simulink model "Sequence_Manager"  (R2024a)
settings: Solver=ode1  StartTime=0.0  StopTime=inf  FixedStep=0.1  RelTol=1e-3
undefined symbols (not defined in the file): Angle, Axis, Battery, s
libraries: robotcorelib x6, eeGeneralControl x6, slpidlib x4
settings Model: Creator=Sasha  LastModifiedBy=Sasha

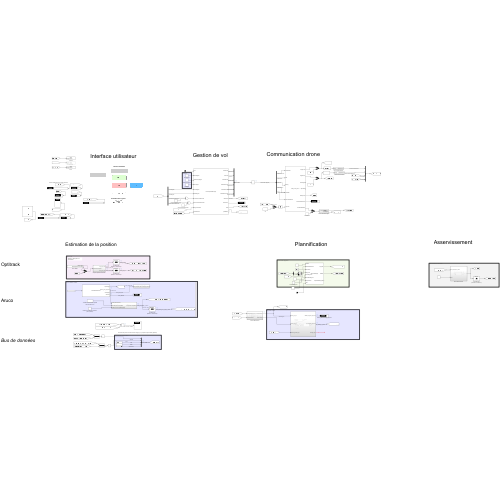
[thumbnail: Simulink's stored preview of the top-level diagram]
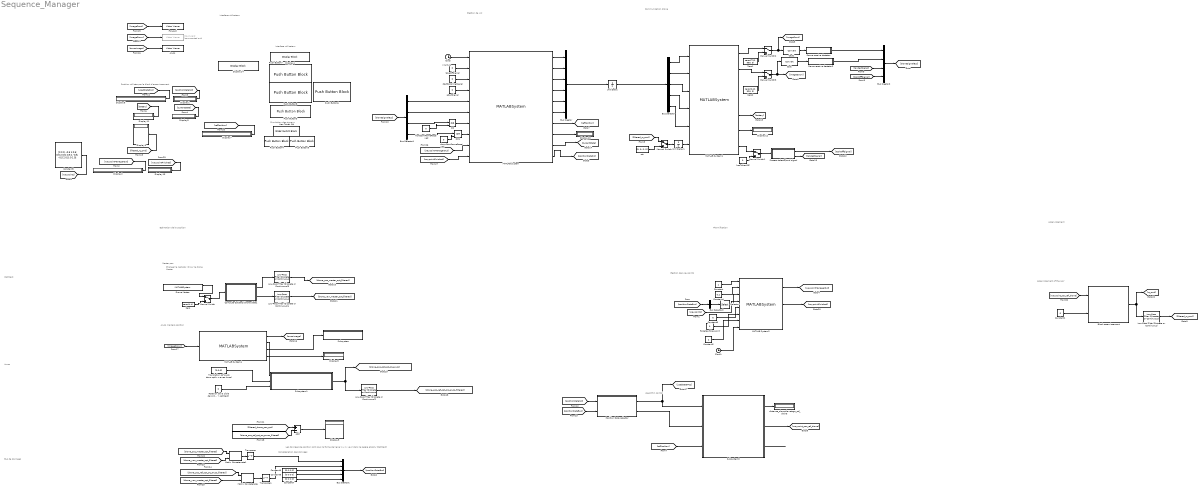
== system Sequence_Manager ==
  note: Plannification
  note: Estimation de la position
  note: Position utilisée par le block d'asservissement
  note: Gestion des waypoints
  note: Interface
  note: Concaténation des données
  note: Les données de position sont sous la forme de ligne (x,y,z, yaw) dans le repère absolu (Optitrack)
  note: Simulation des signaux
  note: Master pos
  note: Changer le rigibody ID sur le drone Master
  note: Algorithm control
  note: Interface utilisateur
  note: Aruco markers position
  note: Optitrack
  note: Aruco
  note: Bus de données
  note: Asservissement
  note: Gestion de vol
  note: Communication drone
  note: Interface utilisateur
  note: Asservissement of the UAV
  Add : Sum  Inputs=+-
  Aruco : VideoViewer  FigPos=[1259 530 247.333333333333 297.333333333333]
  "Block asservissement " : Subsystem
  Bus Creator : BusCreator  Inputs=6
  Bus Creator1 : BusCreator  Inputs=5
  Bus Creator2 : BusCreator  Inputs=4
  Bus Selector : BusSelector  OutputSignals=enableVideoCmd,takeOffCmd,landCmd,enableRcCmd,videoDirectionCmd
  Bus Selector1 : BusSelector  OutputSignals=tookOffSignal,landedSignal,frontCamFrameReceived,downCamFrameReceived
  Bus Selector2 : BusSelector  OutputSignals=Optitrack
  Cast : DataTypeConversion  SaturateOnIntegerOverflow=off  RndMeth=Floor
  Cast1 : DataTypeConversion  SaturateOnIntegerOverflow=off  RndMeth=Floor
  Clock : Clock
  Clock1 : Clock
  Compute Optitrack Drone data1 : Subsystem
  Constant : Constant
  Constant1 : Constant  Value=0
  Constant2 : Constant  Value=2
  Constant4 : Constant  Value=0.2
  Constant5 : Constant  Value="[0 0 0; -0.5 1 0.5;  0.5 2 0.5; 0.5 1 -0.5; -0.5 2 0.5; 0 1 0]"
  Constant6 : Constant  Value=6
  Constant7 : Constant  Value=[0 0 0 0]
  Constant8 : Constant  Value=[0 0 0 0]
  Constant9 : Constant  Value=[0 0 0 0]
  Display{1..3,5..13} (12 alike) : Display
  Display14 : DisplayBlock  LabelPosition=Hide  Format=Custom  Transparency=1  FormatString=Battery : %s/100
  Display4 : DisplayBlock  LabelPosition=Hide  Format=Integer  Transparency=1  FormatString=%s
  Downward : VideoViewer  Commented=on  FigPos=[1261.66666666667 919.333333333333 248 307.333333333333]
  Drone Master : MATLABSystem  System=OptilinkSystem  HostIP=10.147.125.15  ClientIP=10.147.125.17  RigidbodyID=1  SimulateUsing=Interpreted execution
      mask Type: OptilinkSystem
      mask Display:
      | disp('OptilinkSystem');
      | port_label('output',1,'Drones data');
      | port_label('output',2,'Connected');
  Forward : VideoViewer  FigPos=[616.333333333333 756 875.333333333333 522.666666666667]
  Frame receive dectetor : Subsystem
  Frame receive dectetor2 : Subsystem
  Has Taken Off : SliderSwitchBlock
      settings: Values={{'Off', 'On'}, [0 1]}
  Low-Pass Filter (Discrete or Continuous) : eeGeneralControl/Low-Pass Filter (Discrete or Continuous)  K=1  T=1  B=inf  A=-inf  init_option=Inherited from block input  x0=0  Ts=-1
  Low-Pass Filter (Discrete or Continuous)2 : eeGeneralControl/Low-Pass Filter (Discrete or Continuous)  K=1  T=1.5  B=inf  A=-inf  init_option=Inherited from block input  x0=0  Ts=-1
  Low-Pass Filter (Discrete or Continuous)4 : eeGeneralControl/Low-Pass Filter (Discrete or Continuous)  K=1  T=1.5  B=inf  A=-inf  init_option=Inherited from block input  x0=0  Ts=-1
  Low-Pass Filter (Discrete or Continuous)5 : eeGeneralControl/Low-Pass Filter (Discrete or Continuous)  K=1  T=1.5  B=inf  A=-inf  init_option=Inherited from block input  x0=0  Ts=-1
  MATLAB System : MATLABSystem  System=DroneSequenceManager  HomePosition=[ 0, 1.5, 0 ]  SimulateUsing=Code generation
      mask Type: DroneSequenceManager
      mask Display:
      | disp('DroneSequenceManager');
      | port_label('input',1,'time');
      | port_label('input',2,'takeOffSignal');
      | port_label('input',3,'startPatrolingSignal');
      | port_label('input',4,'abortSignal');
      | port_label('input',5,'tookOffSignal');
      | port_label('input',6,'landedSignal');
      | port_label('input',7,'frontCamFrameReceived');
      | port_label('input',8,'downCamFrameReceived');
      | port_label('input',9,'waypointToFollow');
      | port_label('input',10,'finishedFollow');
      | port_label('output',1,'takeoffCmd');
      | port_label('output',2,'landCmd');
      | port_label('output',3,'enableRcCmd');
      | port_label('output',4,'enableVideoCmd');
      | port_label('output',5,'enableSlamCmd');
      | port_label('output',6,'videoDirectionCmd');
      | port_label('output',7,'refPosition');
      | port_label('output',8,'timeCounter');
      | port_label('output',9,'state');
      | port_label('output',10,'posDataSrc');
  MATLAB System1 : MATLABSystem  System=Tello_drone_control  droneIP=127.0.0.1  SimulateUsing=Interpreted execution
      mask Type: Tello_drone_control
      mask Display:
      | disp('Tello_drone_control');
      | port_label('input',1,'enableVideo');
      | port_label('input',2,'tkoff');
      | port_label('input',3,'landing');
      | port_label('input',4,'enableRC');
      | port_label('input',5,'cmdVideoDirection');
      | port_label('input',6,'rcspeeds');
      | port_label('output',1,'imageFront');
      | port_label('output',2,'imageDown');
      | port_label('output',3,'Eulerangles');
      | port_label('output',4,'speedXYZ');
      | port_label('output',5,'batteryLevel');
      | port_label('output',6,'currentVideoDirection');
      | port_label('output',7,'hasTakenOffStatus');
  MATLAB System2 : MATLABSystem  System=WaypointManager  SimulateUsing=Code generation
      mask Type: WaypointManager
      mask Display:
      | disp('WaypointManager');
      | port_label('input',1,'enable');
      | port_label('input',2,'lookaheadDistance');
      | port_label('input',3,'currentPos');
      | port_label('input',4,'waypoints');
      | port_label('input',5,'numWaypoints');
      | port_label('input',6,'forceNextWaypoint');
      | port_label('input',7,'requiredTime');
      | port_label('input',8,'time');
      | port_label('output',1,'waypoint');
      | port_label('output',2,'finished');
      | port_label('output',3,'elapsedTimeWaypoint');
  MATLAB System4 : MATLABSystem  System=ArucoMarkerDetection  markerSizeInMM=150  markerFamily=DICT_4X4_250  maxMarkers=1  focalLength=[222.5, 224]  principalPoint=[156 ,116]  imageSize=[240,320]  SimulateUsing=Interpreted execution
      mask Type: ArucoMarkerDetection
      mask Display:
      | disp('ArucoMarkerDetection');
      | port_label('input',1,'I');
      | port_label('output',1,'outputImage');
      | port_label('output',2,'camera_pos_ref_aruco');
      | port_label('output',3,'eulerAngles');
      | port_label('output',4,'detection');
  Manual Switch{,1..4} (5 alike) : ManualSwitch
  Matrix Concatenate : Concatenate  ConcatenateDimension=2
  Matrix Concatenate1 : Concatenate  ConcatenateDimension=2
  OR : Logic  Operator=OR  IconShape=distinctive  AllPortsSameDT=off  OutDataTypeStr=boolean
  OR1 : Logic  Operator=OR  IconShape=distinctive  AllPortsSameDT=off  OutDataTypeStr=boolean
  Position Data selector : Subsystem
  Process takeoff/land signal : Subsystem
  Push Button3 : PushButtonBlock  ButtonText=Force next waypoint  OffValue=0.000000
  Push Button4 : PushButtonBlock  ButtonText=Front cam received  OffValue=0.000000
  Push Button5 : PushButtonBlock  ButtonText=Down cam received  OffValue=0.000000
  Push Button6 : PushButtonBlock  ButtonText=Start patrol  Opacity=0.8  OffValue=0.000000
  Push Button7 : PushButtonBlock  ButtonText=Décoler  OffValue=0.000000
  Push Button8 : PushButtonBlock  ButtonText=Atterir  OffValue=0.000000
  Rotation de la cible dans Optitrack (Axe Y optitrack) : Constant  Value=0
  Selector : Selector  InputPortWidth=4  IndexOptions=Index vector (dialog)  Indices=[1 2 3]  OutputSizes=1
  Subsystem : Subsystem
  Subsystem1 : Subsystem
  Subsystem3 : Subsystem
  "Translation ref Aruco dans optitrack (dans les axes Aruco) " : Constant  Value=[0;0;0]
  Transpose : Math  Operator=transpose
  Transpose1 : Math  Operator=transpose
  Unit Delay : UnitDelay  SampleTime=-1  HasFrameUpgradeWarning=on
  Unit Delay1 : UnitDelay  InitialCondition=[0,0,0,0]  SampleTime=-1  HasFrameUpgradeWarning=on
  Zero : Constant  Value=zeros(4,4)  OutDataTypeStr=Inherit: Inherit via back propagation
  Zero1 : Constant  Value=zeros(720, 960, 3)  OutDataTypeStr=Inherit: Inherit via back propagation
  Zero2 : Constant  Value=zeros(240, 320, 3)  OutDataTypeStr=Inherit: Inherit via back propagation
  abortSignal : Constant  Value=0
  cst : Constant  Value=[0; 0; 0; 0]
  distance_slave/slavetogo_ref_drone : Display
  downCamFrameReceived : Constant  Value=0
  forceNextWaypoint : Constant  Value=0
  frontCamFrameReceived : Constant  Value=0
  hasTakenOff : Constant  Value=0
  startPatrolingSignal : Constant  Value=0
  takeOffSignal : Constant  Value=0
  wires:
  Clock/1 -> MATLAB System/1
  takeOffSignal/1 -> MATLAB System/2
  MATLAB System/6 -> Bus Creator/6  "videoDirectionCmd"
  Zero2/1 -> Manual Switch3/2
  Frame receive dectetor2/1(frameReceived) -> Bus Creator2/2  "downCamFrameReceived"
  abortSignal/1 -> MATLAB System/4
  Bus Selector1/1 -> MATLAB System/5  "<tookOffSignal>"
  Bus Selector1/2 -> MATLAB System/6  "<landedSignal>"
  MATLAB System/8 -> Display10/1
  Frame receive dectetor/1(frameReceived) -> Bus Creator2/1  "frontCamFrameReceived"
  OR/1 -> MATLAB System/7
  Bus Selector1/3 -> OR/1  "<frontCamFrameReceived>"
  frontCamFrameReceived/1 -> OR/2
  OR1/1 -> MATLAB System/8
  Bus Selector1/4 -> OR1/1  "<downCamFrameReceived>"
  downCamFrameReceived/1 -> OR1/2
  MATLAB System/1 -> Bus Creator/1  "takeOffCmd"
  MATLAB System/2 -> Bus Creator/2  "landCmd"
  MATLAB System/3 -> Bus Creator/3  "enableRcCmd"
  MATLAB System/4 -> Bus Creator/4  "enableVideoCmd"
  MATLAB System/5 -> Bus Creator/5  "enableSlamCmd"
  MATLAB System/9 -> [currentState]
  startPatrolingSignal/1 -> MATLAB System/3
  Constant9/1 -> Bus Creator1/3  "IMU"
  MATLAB System/10 -> [positionDataSrc]
  Constant4/1 -> MATLAB System2/2
  Bus Selector2/1 -> Selector/1  "<Optitrack>"
  [waypoints] -> MATLAB System2/4
  Constant6/1 -> MATLAB System2/5
  MATLAB System2/1 -> [waypointManagerOut]
  Drone Master/1 -> Manual Switch/1
  Compute Optitrack Drone data1/1(drone_pos_opt) -> Low-Pass Filter (Discrete or Continuous)5/1  "drone_pos_ref_opt"
  Low-Pass Filter (Discrete or Continuous)4/1 -> [drone_yaw_master_opt_filtered]  "drone_yaw_opt"
  Compute Optitrack Drone data1/2(drone_yaw_opt) -> Low-Pass Filter (Discrete or Continuous)4/1  "drone_yaw_ref_opt"
  Low-Pass Filter (Discrete or Continuous)5/1 -> [drone_pos_master_opt_filtered]  "drone_pos_opt"
  MATLAB System1/5 -> [battery]
  MATLAB System1/6 -> Display12/1
  Subsystem3/3(Consigne_yaw) -> ?
  Subsystem3/2(pos_waypoint_ref_drone) -> [waypoint_pos_ref_drone]  "pos_slavetogo_ref_drone"
  Position Data selector/2(Drone Yaw Opt) -> Subsystem3/2(drone_yaw_opt)
  Subsystem3/1(distance_waypoint_ref_drone) -> distance_slave/slavetogo_ref_drone/1
  [refPosition] -> Subsystem3/3(reference_position_opt)
  [filtered_rc_cmd] -> Manual Switch4/1  "filtered_rc_cmd"
  Manual Switch/1 -> Compute Optitrack Drone data1/1(Optitrack Drone TForm)
  Zero/1 -> Manual Switch/2
  Bus Creator/1 -> Unit Delay/1  "droneCmdBus"
  Bus Selector/2 -> MATLAB System1/2  "<takeOffCmd>"
  Bus Selector/3 -> MATLAB System1/3  "<landCmd>"
  Bus Selector/1 -> MATLAB System1/1  "<enableVideoCmd>"
  Bus Selector/4 -> MATLAB System1/4  "<enableRcCmd>"
  Bus Creator1/1 -> [positionDataBus]  "positionDataBus"
  Bus Selector/5 -> MATLAB System1/5  "<videoDirectionCmd>"
  Constant7/1 -> Bus Creator1/5  "SensorFusion"
  Constant8/1 -> Bus Creator1/4  "SLAM"
  hasTakenOff/1 -> Manual Switch1/2
  Constant/1 -> MATLAB System2/1
  [landedSignal] -> Bus Creator2/3  "landedSignal"
  [tookOfffSignal] -> Bus Creator2/4  "tookOffSignal"
  Bus Creator2/1 -> [droneSignalBus]
  [droneSignalBus] -> Bus Selector1/1
  MATLAB System/7 -> [refPosition]  "refPosition"
  Matrix Concatenate1/1 -> Transpose/1
  [positionDataBus] -> Bus Selector2/1
  Constant5/1 -> [waypoints]
  [waypointManagerOut] -> Display2/1
  [currentState] -> Display5/1
  [positionDataSrc] -> Display1/1
  [usedDataPos] -> Display6/1
  [positionDataSrc] -> Position Data selector/1(Position Data Source)
  [positionDataBus] -> Position Data selector/2(Position Data Bus)
  Position Data selector/1(Drone Position Opt) -> Subsystem3/1(drone_pos_opt), [usedDataPos]  "measured_pos"
  MATLAB System1/7 -> Manual Switch1/1
  MATLAB System1/2 -> Manual Switch3/1
  Manual Switch3/1 -> [imageDown], Cast/1
  Zero1/1 -> Manual Switch2/2
  MATLAB System1/1 -> Manual Switch2/1
  Manual Switch4/1 -> Unit Delay1/1
  cst/1 -> Manual Switch4/2
  Manual Switch2/1 -> [imageFront], Cast1/1
  Unit Delay/1 -> Bus Selector/1  "droneCmdBus (delayed)"
  [imageDown] -> Downward/1
  [imageFront] -> Forward/1
  Cast/1 -> Frame receive dectetor2/1(image)
  Cast1/1 -> Frame receive dectetor/1(image)
  [arucoImage] -> Aruco/1
  Unit Delay1/1 -> MATLAB System1/6
  Manual Switch1/1 -> Process takeoff/land signal/1("hasTakenOffStatus ")
  Process takeoff/land signal/1(tookOffSignal) -> [tookOfffSignal]
  Process takeoff/land signal/2(landedSignal) -> [landedSignal]
  [battery] -> Display11/1
  [filtered_rc_cmd] -> Display3/1
  forceNextWaypoint/1 -> MATLAB System2/6
  [refPosition] -> Display7/1
  Matrix Concatenate/1 -> Transpose1/1  "Aruco"
  Transpose/1 -> Bus Creator1/1  "Optitrack"
  Selector/1 -> MATLAB System2/3
  MATLAB System4/2 -> Subsystem1/1(Drone position ref Aruco)  "raw_aruco_pos"
  MATLAB System4/1 -> [arucoImage]
  [imageDown] -> MATLAB System4/1
  Subsystem1/1(Drone position ref Optitrack) -> Low-Pass Filter (Discrete or Continuous)2/1, [drone_pos_ref_opt_src_aruco]  "drone_pos_ref_opt_src_aruco"
  Add/1 -> Display9/1  "err_pos_aruco_optitrack"
  Low-Pass Filter (Discrete or Continuous)2/1 -> [drone_pos_ref_opt_src_aruco_filtered]  "filtered_drone_pos_ref_opt_src_aruco"
  MATLAB System4/4 -> Display8/1  "aruco_detection"
  "Translation ref Aruco dans optitrack (dans les axes Aruco) "/1 -> Subsystem1/2(Translation Aruco ref Optitrack)
  MATLAB System4/3 -> Subsystem/1(dro_euler_ZYX_aruco)  "aruco_euler_ZYX"
  [filtered_drone_pos_opt] -> Add/1
  Rotation de la cible dans Optitrack (Axe Y optitrack)/1 -> Subsystem1/3(Rotation sur axe Y Optitrack (alpha))
  [drone_pos_ref_opt_src_aruco_filtered] -> Add/2
  [drone_yaw_master_opt_filtered] -> Matrix Concatenate1/2
  [drone_pos_master_opt_filtered] -> Matrix Concatenate1/1
  [drone_pos_ref_opt_src_aruco_filtered] -> Matrix Concatenate/1
  Transpose1/1 -> Bus Creator1/2  "Aruco"
  [drone_yaw_master_opt_filtered] -> Matrix Concatenate/2
  MATLAB System2/2 -> [waypointFinished]
  [waypointManagerOut] -> MATLAB System/9
  [waypointFinished] -> MATLAB System/10
  "Block asservissement "/1(Out1) -> [rc_cmd], Low-Pass Filter (Discrete or Continuous)/1
  Constant1/1 -> "Block asservissement "/2(yaw)
  [waypoint_pos_ref_drone] -> "Block asservissement "/1(pos_waypoint_ref_drone)
  [waypointFinished] -> Display13/1
  Constant2/1 -> MATLAB System2/7
  Clock1/1 -> MATLAB System2/8
  Low-Pass Filter (Discrete or Continuous)/1 -> [filtered_rc_cmd]

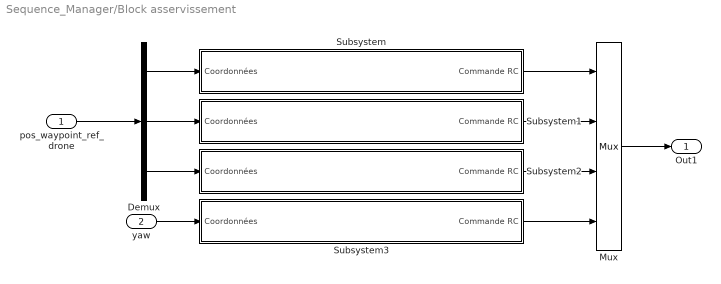
== system Sequence_Manager/Block asservissement  ==
  pos_waypoint_ref_drone : Inport
  yaw : Inport  Port=2
  Demux : Demux  Outputs=3
  Mux : Mux
  Subsystem : Subsystem
  Subsystem1 : Subsystem
  Subsystem2 : Subsystem
  Subsystem3 : Subsystem
  Out1 : Outport
  wires:
  pos_waypoint_ref_drone/1 -> Demux/1
  Mux/1 -> Out1/1
  Demux/1 -> Subsystem/1(Coordonnées)
  Subsystem/1(Commande RC) -> Mux/1
  Subsystem1/1(Commande RC) -> Mux/2
  Demux/2 -> Subsystem1/1(Coordonnées)
  Demux/3 -> Subsystem2/1(Coordonnées)
  Subsystem2/1(Commande RC) -> Mux/3
  yaw/1 -> Subsystem3/1(Coordonnées)
  Subsystem3/1(Commande RC) -> Mux/4

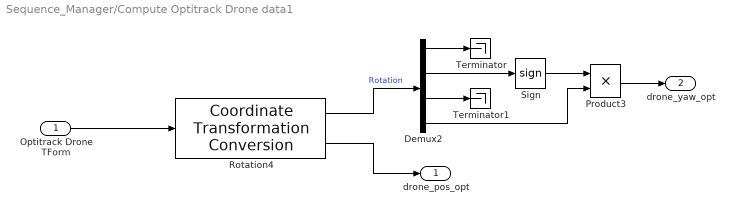
== system Sequence_Manager/Compute Optitrack Drone data1 ==
  Optitrack Drone TForm : Inport
  Demux2 : Demux
  Product3 : Product
  Rotation4 : robotcorelib/Coordinate Transformation Conversion  InputRepresentation=Homogeneous Transformation  InputEulerSequence=XYZ  ShowTrVecInputPort=on  OutputRepresentation=Axis-Angle  OutputEulerSequence=XYZ  ShowTrVecOutputPort=on  SimulateUsing=Code generation
      settings: LibrarySourceBlock=uavutilslib/Coordinate Transformation Conversion
  Sign : Signum
  Terminator : Terminator
  Terminator1 : Terminator
  drone_pos_opt : Outport
  drone_yaw_opt : Outport  Port=2
  wires:
  Rotation4/2 -> drone_pos_opt/1
  Demux2/4 -> Product3/2
  Rotation4/1 -> Demux2/1  "Rotation"
  Sign/1 -> Product3/1
  Demux2/2 -> Sign/1
  Product3/1 -> drone_yaw_opt/1
  Optitrack Drone TForm/1 -> Rotation4/1
  Demux2/3 -> Terminator1/1
  Demux2/1 -> Terminator/1

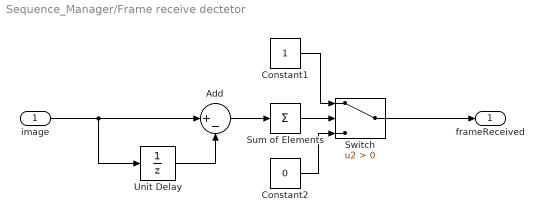
== system Sequence_Manager/Frame receive dectetor ==
  image : Inport
  Add : Sum  Inputs=|+-
  Constant1 : Constant
  Constant2 : Constant  Value=0
  Sum of Elements : Sum  Inputs=+
  Switch : Switch  Criteria=u2 > Threshold  SaturateOnIntegerOverflow=off  InputSameDT=off
  Unit Delay : UnitDelay  SampleTime=-1  HasFrameUpgradeWarning=on
  frameReceived : Outport
  wires:
  Switch/1 -> frameReceived/1
  Constant1/1 -> Switch/1
  image/1 -> Add/1, Unit Delay/1
  Unit Delay/1 -> Add/2
  Add/1 -> Sum of Elements/1
  Sum of Elements/1 -> Switch/2
  Constant2/1 -> Switch/3

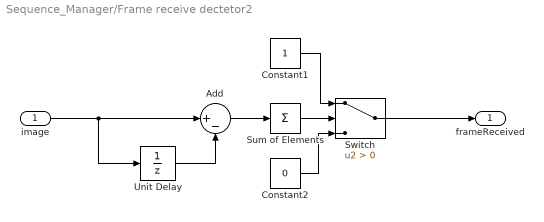
== system Sequence_Manager/Frame receive dectetor2 ==
  image : Inport
  Add : Sum  Inputs=|+-
  Constant1 : Constant
  Constant2 : Constant  Value=0
  Sum of Elements : Sum  Inputs=+
  Switch : Switch  Criteria=u2 > Threshold  SaturateOnIntegerOverflow=off  InputSameDT=off
  Unit Delay : UnitDelay  SampleTime=-1  HasFrameUpgradeWarning=on
  frameReceived : Outport
  wires:
  Switch/1 -> frameReceived/1
  Constant1/1 -> Switch/1
  image/1 -> Add/1, Unit Delay/1
  Unit Delay/1 -> Add/2
  Add/1 -> Sum of Elements/1
  Sum of Elements/1 -> Switch/2
  Constant2/1 -> Switch/3

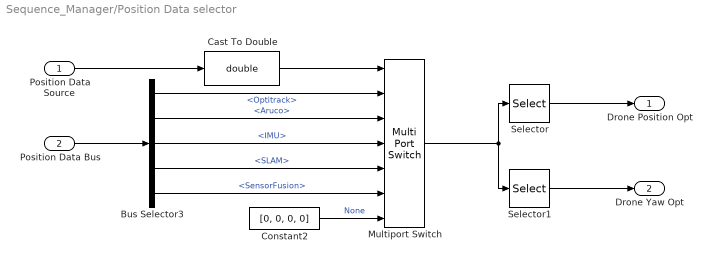
== system Sequence_Manager/Position Data selector ==
  Position Data Source : Inport
  Position Data Bus : Inport  Port=2
  Bus Selector3 : BusSelector  OutputSignals=Optitrack,Aruco,IMU,SLAM,SensorFusion
  Cast To Double : DataTypeConversion  OutDataTypeStr=double  SaturateOnIntegerOverflow=off  RndMeth=Floor
  Constant2 : Constant  Value=[0, 0, 0, 0]
  Multiport Switch : MultiPortSwitch  DataPortOrder=Specify indices  Inputs=6  DataPortIndices={2,3,4,5,6,1}  DiagnosticForDefault=None  SaturateOnIntegerOverflow=off  InputSameDT=off
  Selector : Selector  InputPortWidth=4  IndexOptions=Index vector (dialog)  Indices=[1 2 3]  OutputSizes=1
  Selector1 : Selector  InputPortWidth=4  IndexOptions=Index vector (dialog)  Indices=[4]  OutputSizes=1
  Drone Position Opt : Outport
  Drone Yaw Opt : Outport  Port=2
  wires:
  Multiport Switch/1 -> Selector/1, Selector1/1
  Position Data Source/1 -> Cast To Double/1
  Constant2/1 -> Multiport Switch/7  "None"
  Bus Selector3/3 -> Multiport Switch/4  "<IMU>"
  Bus Selector3/2 -> Multiport Switch/3  "<Aruco>"
  Bus Selector3/5 -> Multiport Switch/6  "<SensorFusion>"
  Bus Selector3/4 -> Multiport Switch/5  "<SLAM>"
  Cast To Double/1 -> Multiport Switch/1
  Bus Selector3/1 -> Multiport Switch/2  "<Optitrack>"
  Position Data Bus/1 -> Bus Selector3/1
  Selector/1 -> Drone Position Opt/1
  Selector1/1 -> Drone Yaw Opt/1

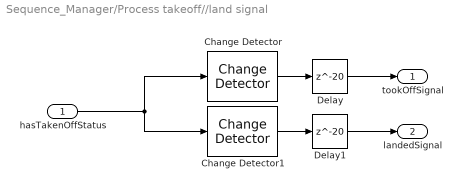
== system Sequence_Manager/Process takeoff//land signal ==
  "hasTakenOffStatus " : Inport
  Change Detector : eeGeneralControl/Change Detector  VariantControl=Variant1  LabelModeActiveChoice=Discrete  ChangeType=Rising edge  x0=0  Ts=-1
      settings: LibrarySourceBlock=ee_sl_lib/General Control/Change Detector
  Change Detector1 : eeGeneralControl/Change Detector  VariantControl=Variant1  LabelModeActiveChoice=Discrete  ChangeType=Falling edge  x0=0  Ts=-1
      settings: LibrarySourceBlock=ee_sl_lib/General Control/Change Detector
  Delay : Delay  DelayLength=20
  Delay1 : Delay  DelayLength=20
  tookOffSignal : Outport
  landedSignal : Outport  Port=2
  wires:
  Change Detector/1 -> Delay/1
  "hasTakenOffStatus "/1 -> Change Detector1/1, Change Detector/1
  Change Detector1/1 -> Delay1/1
  Delay1/1 -> landedSignal/1
  Delay/1 -> tookOffSignal/1

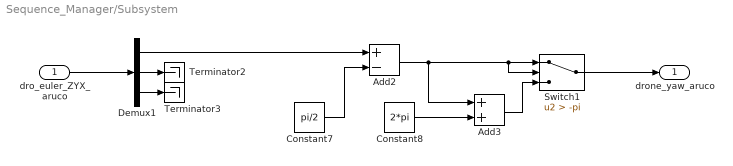
== system Sequence_Manager/Subsystem ==
  dro_euler_ZYX_aruco : Inport
  Add2 : Sum  Inputs=+-
  Add3 : Sum
  Constant7 : Constant  Value=pi/2
  Constant8 : Constant  Value=2*pi
  Demux1 : Demux  Outputs=3
  Switch1 : Switch  Criteria=u2 > Threshold  Threshold=-pi  SaturateOnIntegerOverflow=off  InputSameDT=off
  Terminator2 : Terminator
  Terminator3 : Terminator
  drone_yaw_aruco : Outport
  wires:
  dro_euler_ZYX_aruco/1 -> Demux1/1
  Add2/1 -> Add3/1, Switch1/2, Switch1/1
  Demux1/3 -> Terminator3/1
  Constant8/1 -> Add3/2
  Demux1/1 -> Add2/1
  Add3/1 -> Switch1/3
  Constant7/1 -> Add2/2
  Demux1/2 -> Terminator2/1
  Switch1/1 -> drone_yaw_aruco/1

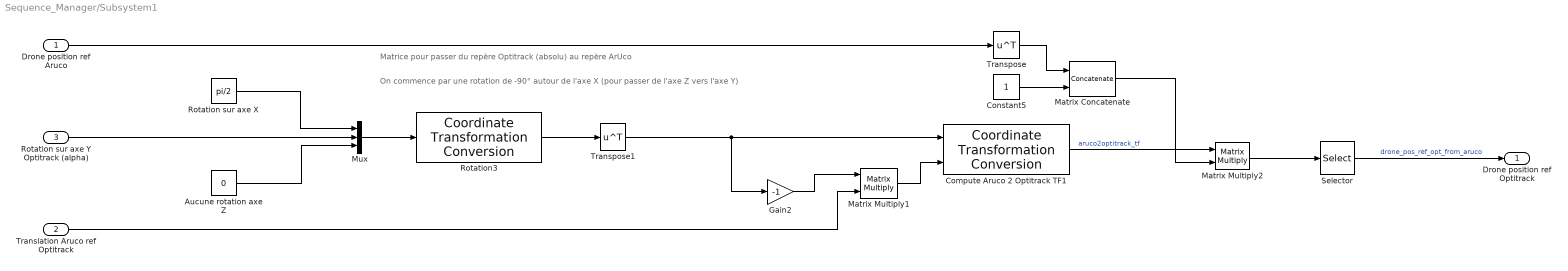
== system Sequence_Manager/Subsystem1 ==
  note: Matrice pour passer du repère Optitrack (absolu) au repère ArUco
  note: On commence par une rotation de -90° autour de l'axe X (pour passer de l'axe Z vers l'axe Y)
  Drone position ref Aruco : Inport
  Translation Aruco ref Optitrack : Inport  Port=2
  Rotation sur axe Y Optitrack (alpha) : Inport  Port=3
  Aucune rotation axe Z : Constant  Value=0
  Compute Aruco 2 Optitrack TF1 : robotcorelib/Coordinate Transformation Conversion  InputRepresentation=Rotation Matrix  InputEulerSequence=XYZ  ShowTrVecInputPort=on  OutputRepresentation=Homogeneous Transformation  OutputEulerSequence=XYZ  ShowTrVecOutputPort=on  SimulateUsing=Code generation
      settings: LibrarySourceBlock=uavutilslib/Coordinate Transformation Conversion
  Constant5 : Constant
  Gain2 : Gain  Gain=-1
  Matrix Concatenate : Concatenate  ConcatenateDimension=2
  Matrix Multiply1 : Product  Multiplication=Matrix(*)
  Matrix Multiply2 : Product  Multiplication=Matrix(*)
  Mux : Mux  Inputs=3
  Rotation sur axe X : Constant  Value=pi/2
  Rotation3 : robotcorelib/Coordinate Transformation Conversion  InputRepresentation=Euler Angles  InputEulerSequence=XYZ  ShowTrVecInputPort=on  OutputRepresentation=Rotation Matrix  OutputEulerSequence=XYZ  ShowTrVecOutputPort=on  SimulateUsing=Code generation
      settings: LibrarySourceBlock=uavutilslib/Coordinate Transformation Conversion
  Selector : Selector  InputPortWidth=4  IndexOptions=Index vector (dialog)  Indices=[1 2 3]  OutputSizes=1
  Transpose : Math  Operator=transpose
  Transpose1 : Math  Operator=transpose
  Drone position ref Optitrack : Outport
  wires:
  Rotation sur axe Y Optitrack (alpha)/1 -> Mux/2
  Transpose/1 -> Matrix Concatenate/1
  Mux/1 -> Rotation3/1
  Constant5/1 -> Matrix Concatenate/2
  Gain2/1 -> Matrix Multiply1/1
  Rotation3/1 -> Transpose1/1
  Matrix Multiply1/1 -> Compute Aruco 2 Optitrack TF1/2
  Rotation sur axe X/1 -> Mux/1
  Transpose1/1 -> Gain2/1, Compute Aruco 2 Optitrack TF1/1
  Matrix Concatenate/1 -> Matrix Multiply2/2
  Aucune rotation axe Z/1 -> Mux/3
  Compute Aruco 2 Optitrack TF1/1 -> Matrix Multiply2/1  "aruco2optitrack_tf"
  Matrix Multiply2/1 -> Selector/1
  Selector/1 -> Drone position ref Optitrack/1  "drone_pos_ref_opt_from_aruco"
  Drone position ref Aruco/1 -> Transpose/1
  Translation Aruco ref Optitrack/1 -> Matrix Multiply1/2

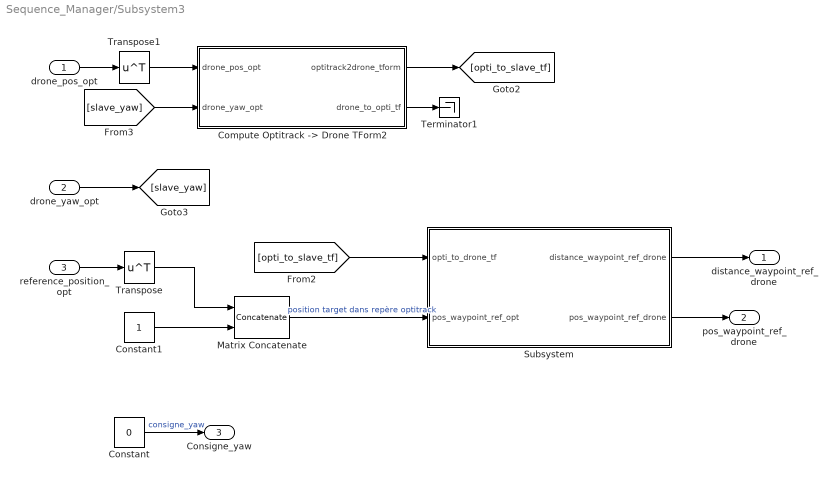
== system Sequence_Manager/Subsystem3 ==
  drone_pos_opt : Inport
  drone_yaw_opt : Inport  Port=2
  reference_position_opt : Inport  Port=3
  "Compute Optitrack -> Drone TForm2" : Subsystem
  Constant : Constant  Value=0
  Constant1 : Constant
  Matrix Concatenate : Concatenate  ConcatenateDimension=2
  Subsystem : Subsystem
  Terminator1 : Terminator
  Transpose : Math  Operator=transpose
  Transpose1 : Math  Operator=transpose
  distance_waypoint_ref_drone : Outport
  pos_waypoint_ref_drone : Outport  Port=2
  Consigne_yaw : Outport  Port=3
  wires:
  Subsystem/1(distance_waypoint_ref_drone) -> distance_waypoint_ref_drone/1
  Subsystem/2(pos_waypoint_ref_drone) -> pos_waypoint_ref_drone/1
  Constant/1 -> Consigne_yaw/1  "consigne_yaw"
  Matrix Concatenate/1 -> Subsystem/2(pos_waypoint_ref_opt)  "position target dans repère optitrack"
  "Compute Optitrack -> Drone TForm2"/2(drone_to_opti_tf) -> Terminator1/1
  [slave_yaw] -> "Compute Optitrack -> Drone TForm2"/2(drone_yaw_opt)
  drone_pos_opt/1 -> Transpose1/1
  drone_yaw_opt/1 -> [slave_yaw]
  "Compute Optitrack -> Drone TForm2"/1(optitrack2drone_tform) -> [opti_to_slave_tf]
  [opti_to_slave_tf] -> Subsystem/1(opti_to_drone_tf)
  Transpose/1 -> Matrix Concatenate/1
  Constant1/1 -> Matrix Concatenate/2
  reference_position_opt/1 -> Transpose/1
  Transpose1/1 -> "Compute Optitrack -> Drone TForm2"/1(drone_pos_opt)

== system Sequence_Manager/Block asservissement /Subsystem ==
  Coordonnées : Inport
  Abs : Abs  SaturateOnIntegerOverflow=off
  Constant : Constant  Value=0
  PID Controller4 : slpidlib/PID Controller  Controller=P  Form=Parallel  TimeDomain=Discrete-time  UseExternalTs=off  SampleTime=-1  IntegratorMethod=Forward Euler  FilterMethod=Forward Euler  ControllerParametersSource=internal  P=30  I=0.0168470505938331  UseKiTs=off  D=0.181138103439247  UseExternalDerivativeSource=off  N=1.15322702769143  UseFilter=on  TunerSelectOption=Transfer Function Based (PID Tuner App)  InitialConditionSource=internal  InitialConditionForIntegrator=0  InitialConditionForFilter=0  DifferentiatorICPrevScaledInput=0  ExternalReset=none  TrackingMode=off  Kt=1  LimitOutput=off  SatLimitsSource=internal  UpperSaturationLimit=inf  LowerSaturationLimit=-inf  LinearizeAsGain=on  AntiWindupMode=none  Kb=1  LimitIntegrator=on  UpperIntegratorSaturationLimit=0.5  LowerIntegratorSaturationLimit=-0.5  POutMin=[]  POutMax=[]  IOutMin=[]  IOutMax=[]  DOutMin=[]  DOutMax=[]  NOutMin=[]  NOutMax=[]  SumOutMin=[]  SumOutMax=[]  SaturationOutMin=[]  SaturationOutMax=[]  PParamMin=[]  PParamMax=[]  IParamMin=[]  IParamMax=[]  DParamMin=[]  DParamMax=[]  NParamMin=[]  NParamMax=[]  KbParamMin=[]  KbParamMax=[]  KtParamMin=[]  KtParamMax=[]  KbOutMin=[]  KbOutMax=[]  KtOutMin=[]  KtOutMax=[]  IntegratorOutMin=[]  IntegratorOutMax=[]  FilterOutMin=[]  FilterOutMax=[]  SumI1OutMin=[]  SumI1OutMax=[]  SumI2OutMin=[]  SumI2OutMax=[]  SumI3OutMin=[]  SumI3OutMax=[]  SumI4OutMin=[]  SumI4OutMax=[]  SumDOutMin=[]  SumDOutMax=[]  DifferentiatorOutMin=[]  DifferentiatorOutMax=[]  FilterDiffOutCoefMin=[]  FilterDiffOutCoefMax=[]  ReciprocalOutMin=[]  ReciprocalOutMax=[]  SumDenOutMin=[]  SumDenOutMax=[]  SumNumOutMin=[]  SumNumOutMax=[]  DivideOutMin=[]  DivideOutMax=[]  UdiffTsProdOutMin=[]  UdiffTsProdOutMax=[]  NTsProdOutMin=[]  NTsProdOutMax=[]  UintegralTsProdOutMin=[]  UintegralTsProdOutMax=[]  UngainTsProdOutMin=[]  UngainTsProdOutMax=[]  ClampingZeroOutDataTypeStr=Inherit: Inherit via back propagation  ClampingZeroOutMin=[]  ClampingZeroOutMax=[]  FilterDenConstantOutDataTypeStr=Inherit: Inherit via back propagation  FilterDenConstantOutMin=[]  FilterDenConstantOutMax=[]  PCopyOutDataTypeStr=Inherit: Inherit via back propagation  PCopyOutMin=[]  PCopyOutMax=[]  NCopyOutDataTypeStr=Inherit: Inherit via back propagation  NCopyOutMin=[]  NCopyOutMax=[]  IntegratorContinuousStateAttributes=''  IntegratorStateMustResolveToSignalObject=off  IntegratorRTWStateStorageClass=Auto  FilterContinuousStateAttributes=''  FilterStateMustResolveToSignalObject=off  FilterRTWStateStorageClass=Auto  ParallelPVariant=InternalParameters  IdealPVariant=Disabled  IVariant=Disabled  DVariant=Disabled  IntegratorVariant=Disabled  SatVariant=Disabled  AWVariant=Disabled  PCopyVariant=Disabled  TRVariant=Disabled  FdbkBlocksVariant=Forward  IdealPFdbkVariant=Disabled  SatFdbkVariant=Disabled  DerivativeFilterVariant=Disabled  NVariant=Disabled  NCopyVariant=Disabled_SignalSpec  FilterICVariant=Disabled  IntegratorICVariant=Disabled  ExternalResetVariant=Disabled  TRSumVariant=Passthrough  SumFdbkVariant=Disabled  SumVariant=Passthrough_P  TsampFilterVariant=InternalTs  TsampNgainVariant=Passthrough  TsampIntegralVariant=Disabled_SignalSpec  ExternalSaturationOutDataTypeStr=Inherit: Same as second input  DerivativeSourceVariant=Disabled
  Saturation : Saturate  UpperLimit=30  LowerLimit=-30
  Switch : Switch  Criteria=u2 > Threshold  Threshold=0.01  SaturateOnIntegerOverflow=off  InputSameDT=off
  Commande RC : Outport
  wires:
  PID Controller4/1 -> Saturation/1
  Coordonnées/1 -> Abs/1, PID Controller4/1
  Saturation/1 -> Switch/1
  Constant/1 -> Switch/3
  Switch/1 -> Commande RC/1
  Abs/1 -> Switch/2

== system Sequence_Manager/Block asservissement /Subsystem1 ==
  Coordonnées : Inport
  Abs : Abs  SaturateOnIntegerOverflow=off
  Constant : Constant  Value=0
  PID Controller5 : slpidlib/PID Controller  Controller=P  Form=Parallel  TimeDomain=Discrete-time  UseExternalTs=off  SampleTime=-1  IntegratorMethod=Forward Euler  FilterMethod=Forward Euler  ControllerParametersSource=internal  P=30  I=0.0168470505938331  UseKiTs=off  D=0.181138103439247  UseExternalDerivativeSource=off  N=1.15322702769143  UseFilter=on  TunerSelectOption=Transfer Function Based (PID Tuner App)  InitialConditionSource=internal  InitialConditionForIntegrator=0  InitialConditionForFilter=0  DifferentiatorICPrevScaledInput=0  ExternalReset=none  TrackingMode=off  Kt=1  LimitOutput=off  SatLimitsSource=internal  UpperSaturationLimit=inf  LowerSaturationLimit=-inf  LinearizeAsGain=on  AntiWindupMode=none  Kb=1  LimitIntegrator=on  UpperIntegratorSaturationLimit=0.5  LowerIntegratorSaturationLimit=-0.5  POutMin=[]  POutMax=[]  IOutMin=[]  IOutMax=[]  DOutMin=[]  DOutMax=[]  NOutMin=[]  NOutMax=[]  SumOutMin=[]  SumOutMax=[]  SaturationOutMin=[]  SaturationOutMax=[]  PParamMin=[]  PParamMax=[]  IParamMin=[]  IParamMax=[]  DParamMin=[]  DParamMax=[]  NParamMin=[]  NParamMax=[]  KbParamMin=[]  KbParamMax=[]  KtParamMin=[]  KtParamMax=[]  KbOutMin=[]  KbOutMax=[]  KtOutMin=[]  KtOutMax=[]  IntegratorOutMin=[]  IntegratorOutMax=[]  FilterOutMin=[]  FilterOutMax=[]  SumI1OutMin=[]  SumI1OutMax=[]  SumI2OutMin=[]  SumI2OutMax=[]  SumI3OutMin=[]  SumI3OutMax=[]  SumI4OutMin=[]  SumI4OutMax=[]  SumDOutMin=[]  SumDOutMax=[]  DifferentiatorOutMin=[]  DifferentiatorOutMax=[]  FilterDiffOutCoefMin=[]  FilterDiffOutCoefMax=[]  ReciprocalOutMin=[]  ReciprocalOutMax=[]  SumDenOutMin=[]  SumDenOutMax=[]  SumNumOutMin=[]  SumNumOutMax=[]  DivideOutMin=[]  DivideOutMax=[]  UdiffTsProdOutMin=[]  UdiffTsProdOutMax=[]  NTsProdOutMin=[]  NTsProdOutMax=[]  UintegralTsProdOutMin=[]  UintegralTsProdOutMax=[]  UngainTsProdOutMin=[]  UngainTsProdOutMax=[]  ClampingZeroOutDataTypeStr=Inherit: Inherit via back propagation  ClampingZeroOutMin=[]  ClampingZeroOutMax=[]  FilterDenConstantOutDataTypeStr=Inherit: Inherit via back propagation  FilterDenConstantOutMin=[]  FilterDenConstantOutMax=[]  PCopyOutDataTypeStr=Inherit: Inherit via back propagation  PCopyOutMin=[]  PCopyOutMax=[]  NCopyOutDataTypeStr=Inherit: Inherit via back propagation  NCopyOutMin=[]  NCopyOutMax=[]  IntegratorContinuousStateAttributes=''  IntegratorStateMustResolveToSignalObject=off  IntegratorRTWStateStorageClass=Auto  FilterContinuousStateAttributes=''  FilterStateMustResolveToSignalObject=off  FilterRTWStateStorageClass=Auto  ParallelPVariant=InternalParameters  IdealPVariant=Disabled  IVariant=Disabled  DVariant=Disabled  IntegratorVariant=Disabled  SatVariant=Disabled  AWVariant=Disabled  PCopyVariant=Disabled  TRVariant=Disabled  FdbkBlocksVariant=Forward  IdealPFdbkVariant=Disabled  SatFdbkVariant=Disabled  DerivativeFilterVariant=Disabled  NVariant=Disabled  NCopyVariant=Disabled_SignalSpec  FilterICVariant=Disabled  IntegratorICVariant=Disabled  ExternalResetVariant=Disabled  TRSumVariant=Passthrough  SumFdbkVariant=Disabled  SumVariant=Passthrough_P  TsampFilterVariant=InternalTs  TsampNgainVariant=Passthrough  TsampIntegralVariant=Disabled_SignalSpec  ExternalSaturationOutDataTypeStr=Inherit: Same as second input  DerivativeSourceVariant=Disabled
  Saturation1 : Saturate  UpperLimit=30  LowerLimit=-30
  Switch : Switch  Criteria=u2 > Threshold  Threshold=0.01  SaturateOnIntegerOverflow=off  InputSameDT=off
  Commande RC : Outport
  wires:
  Constant/1 -> Switch/3
  Switch/1 -> Commande RC/1
  PID Controller5/1 -> Saturation1/1
  Coordonnées/1 -> Abs/1, PID Controller5/1
  Saturation1/1 -> Switch/1
  Abs/1 -> Switch/2

== system Sequence_Manager/Block asservissement /Subsystem2 ==
  Coordonnées : Inport
  Abs : Abs  SaturateOnIntegerOverflow=off
  Constant : Constant  Value=0
  PID Controller3 : slpidlib/PID Controller  Controller=P  Form=Parallel  TimeDomain=Discrete-time  UseExternalTs=off  SampleTime=-1  IntegratorMethod=Forward Euler  FilterMethod=Forward Euler  ControllerParametersSource=internal  P=-25  I=0.0168470505938331  UseKiTs=off  D=0.181138103439247  UseExternalDerivativeSource=off  N=1.15322702769143  UseFilter=on  TunerSelectOption=Transfer Function Based (PID Tuner App)  InitialConditionSource=internal  InitialConditionForIntegrator=0  InitialConditionForFilter=0  DifferentiatorICPrevScaledInput=0  ExternalReset=none  TrackingMode=off  Kt=1  LimitOutput=off  SatLimitsSource=internal  UpperSaturationLimit=inf  LowerSaturationLimit=-inf  LinearizeAsGain=on  AntiWindupMode=none  Kb=1  LimitIntegrator=on  UpperIntegratorSaturationLimit=0.5  LowerIntegratorSaturationLimit=-0.5  POutMin=[]  POutMax=[]  IOutMin=[]  IOutMax=[]  DOutMin=[]  DOutMax=[]  NOutMin=[]  NOutMax=[]  SumOutMin=[]  SumOutMax=[]  SaturationOutMin=[]  SaturationOutMax=[]  PParamMin=[]  PParamMax=[]  IParamMin=[]  IParamMax=[]  DParamMin=[]  DParamMax=[]  NParamMin=[]  NParamMax=[]  KbParamMin=[]  KbParamMax=[]  KtParamMin=[]  KtParamMax=[]  KbOutMin=[]  KbOutMax=[]  KtOutMin=[]  KtOutMax=[]  IntegratorOutMin=[]  IntegratorOutMax=[]  FilterOutMin=[]  FilterOutMax=[]  SumI1OutMin=[]  SumI1OutMax=[]  SumI2OutMin=[]  SumI2OutMax=[]  SumI3OutMin=[]  SumI3OutMax=[]  SumI4OutMin=[]  SumI4OutMax=[]  SumDOutMin=[]  SumDOutMax=[]  DifferentiatorOutMin=[]  DifferentiatorOutMax=[]  FilterDiffOutCoefMin=[]  FilterDiffOutCoefMax=[]  ReciprocalOutMin=[]  ReciprocalOutMax=[]  SumDenOutMin=[]  SumDenOutMax=[]  SumNumOutMin=[]  SumNumOutMax=[]  DivideOutMin=[]  DivideOutMax=[]  UdiffTsProdOutMin=[]  UdiffTsProdOutMax=[]  NTsProdOutMin=[]  NTsProdOutMax=[]  UintegralTsProdOutMin=[]  UintegralTsProdOutMax=[]  UngainTsProdOutMin=[]  UngainTsProdOutMax=[]  ClampingZeroOutDataTypeStr=Inherit: Inherit via back propagation  ClampingZeroOutMin=[]  ClampingZeroOutMax=[]  FilterDenConstantOutDataTypeStr=Inherit: Inherit via back propagation  FilterDenConstantOutMin=[]  FilterDenConstantOutMax=[]  PCopyOutDataTypeStr=Inherit: Inherit via back propagation  PCopyOutMin=[]  PCopyOutMax=[]  NCopyOutDataTypeStr=Inherit: Inherit via back propagation  NCopyOutMin=[]  NCopyOutMax=[]  IntegratorContinuousStateAttributes=''  IntegratorStateMustResolveToSignalObject=off  IntegratorRTWStateStorageClass=Auto  FilterContinuousStateAttributes=''  FilterStateMustResolveToSignalObject=off  FilterRTWStateStorageClass=Auto  ParallelPVariant=InternalParameters  IdealPVariant=Disabled  IVariant=Disabled  DVariant=Disabled  IntegratorVariant=Disabled  SatVariant=Disabled  AWVariant=Disabled  PCopyVariant=Disabled  TRVariant=Disabled  FdbkBlocksVariant=Forward  IdealPFdbkVariant=Disabled  SatFdbkVariant=Disabled  DerivativeFilterVariant=Disabled  NVariant=Disabled  NCopyVariant=Disabled_SignalSpec  FilterICVariant=Disabled  IntegratorICVariant=Disabled  ExternalResetVariant=Disabled  TRSumVariant=Passthrough  SumFdbkVariant=Disabled  SumVariant=Passthrough_P  TsampFilterVariant=InternalTs  TsampNgainVariant=Passthrough  TsampIntegralVariant=Disabled_SignalSpec  ExternalSaturationOutDataTypeStr=Inherit: Same as second input  DerivativeSourceVariant=Disabled
  Saturation4 : Saturate  UpperLimit=30  LowerLimit=-30
  Switch : Switch  Criteria=u2 > Threshold  Threshold=0.01  SaturateOnIntegerOverflow=off  InputSameDT=off
  Commande RC : Outport
  wires:
  Constant/1 -> Switch/3
  Switch/1 -> Commande RC/1
  PID Controller3/1 -> Saturation4/1
  Coordonnées/1 -> Abs/1, PID Controller3/1
  Saturation4/1 -> Switch/1
  Abs/1 -> Switch/2

== system Sequence_Manager/Block asservissement /Subsystem3 ==
  Coordonnées : Inport
  Gain3 : Gain
  PID Controller1 : slpidlib/PID Controller  Controller=P  Form=Parallel  TimeDomain=Continuous-time  UseExternalTs=off  SampleTime=-1  IntegratorMethod=Forward Euler  FilterMethod=Forward Euler  ControllerParametersSource=internal  P=3  I=0.0168470505938331  UseKiTs=off  D=0.181138103439247  UseExternalDerivativeSource=off  N=1.15322702769143  UseFilter=on  TunerSelectOption=Transfer Function Based (PID Tuner App)  InitialConditionSource=internal  InitialConditionForIntegrator=0  InitialConditionForFilter=0  DifferentiatorICPrevScaledInput=0  ExternalReset=none  TrackingMode=off  Kt=1  LimitOutput=off  SatLimitsSource=internal  UpperSaturationLimit=inf  LowerSaturationLimit=-inf  LinearizeAsGain=on  AntiWindupMode=none  Kb=1  LimitIntegrator=on  UpperIntegratorSaturationLimit=0.5  LowerIntegratorSaturationLimit=-0.5  POutMin=[]  POutMax=[]  IOutMin=[]  IOutMax=[]  DOutMin=[]  DOutMax=[]  NOutMin=[]  NOutMax=[]  SumOutMin=[]  SumOutMax=[]  SaturationOutMin=[]  SaturationOutMax=[]  PParamMin=[]  PParamMax=[]  IParamMin=[]  IParamMax=[]  DParamMin=[]  DParamMax=[]  NParamMin=[]  NParamMax=[]  KbParamMin=[]  KbParamMax=[]  KtParamMin=[]  KtParamMax=[]  KbOutMin=[]  KbOutMax=[]  KtOutMin=[]  KtOutMax=[]  IntegratorOutMin=[]  IntegratorOutMax=[]  FilterOutMin=[]  FilterOutMax=[]  SumI1OutMin=[]  SumI1OutMax=[]  SumI2OutMin=[]  SumI2OutMax=[]  SumI3OutMin=[]  SumI3OutMax=[]  SumI4OutMin=[]  SumI4OutMax=[]  SumDOutMin=[]  SumDOutMax=[]  DifferentiatorOutMin=[]  DifferentiatorOutMax=[]  FilterDiffOutCoefMin=[]  FilterDiffOutCoefMax=[]  ReciprocalOutMin=[]  ReciprocalOutMax=[]  SumDenOutMin=[]  SumDenOutMax=[]  SumNumOutMin=[]  SumNumOutMax=[]  DivideOutMin=[]  DivideOutMax=[]  UdiffTsProdOutMin=[]  UdiffTsProdOutMax=[]  NTsProdOutMin=[]  NTsProdOutMax=[]  UintegralTsProdOutMin=[]  UintegralTsProdOutMax=[]  UngainTsProdOutMin=[]  UngainTsProdOutMax=[]  ClampingZeroOutDataTypeStr=Inherit: Inherit via back propagation  ClampingZeroOutMin=[]  ClampingZeroOutMax=[]  FilterDenConstantOutDataTypeStr=Inherit: Inherit via back propagation  FilterDenConstantOutMin=[]  FilterDenConstantOutMax=[]  PCopyOutDataTypeStr=Inherit: Inherit via back propagation  PCopyOutMin=[]  PCopyOutMax=[]  NCopyOutDataTypeStr=Inherit: Inherit via back propagation  NCopyOutMin=[]  NCopyOutMax=[]  IntegratorContinuousStateAttributes=''  IntegratorStateMustResolveToSignalObject=off  IntegratorRTWStateStorageClass=Auto  FilterContinuousStateAttributes=''  FilterStateMustResolveToSignalObject=off  FilterRTWStateStorageClass=Auto  ParallelPVariant=InternalParameters  IdealPVariant=Disabled  IVariant=Disabled  DVariant=Disabled  IntegratorVariant=Disabled  SatVariant=Disabled  AWVariant=Disabled  PCopyVariant=Disabled  TRVariant=Disabled  FdbkBlocksVariant=Forward  IdealPFdbkVariant=Disabled  SatFdbkVariant=Disabled  DerivativeFilterVariant=Disabled  NVariant=Disabled  NCopyVariant=Disabled_SignalSpec  FilterICVariant=Disabled  IntegratorICVariant=Disabled  ExternalResetVariant=Disabled  TRSumVariant=Passthrough  SumFdbkVariant=Disabled  SumVariant=Passthrough_P  TsampFilterVariant=InternalTs  TsampNgainVariant=Passthrough  TsampIntegralVariant=Disabled_SignalSpec  ExternalSaturationOutDataTypeStr=Inherit: Same as second input  DerivativeSourceVariant=Disabled
  Saturation3 : Saturate  UpperLimit=50  LowerLimit=-50
  Commande RC : Outport
  wires:
  Saturation3/1 -> Commande RC/1
  Gain3/1 -> Saturation3/1
  PID Controller1/1 -> Gain3/1
  Coordonnées/1 -> PID Controller1/1

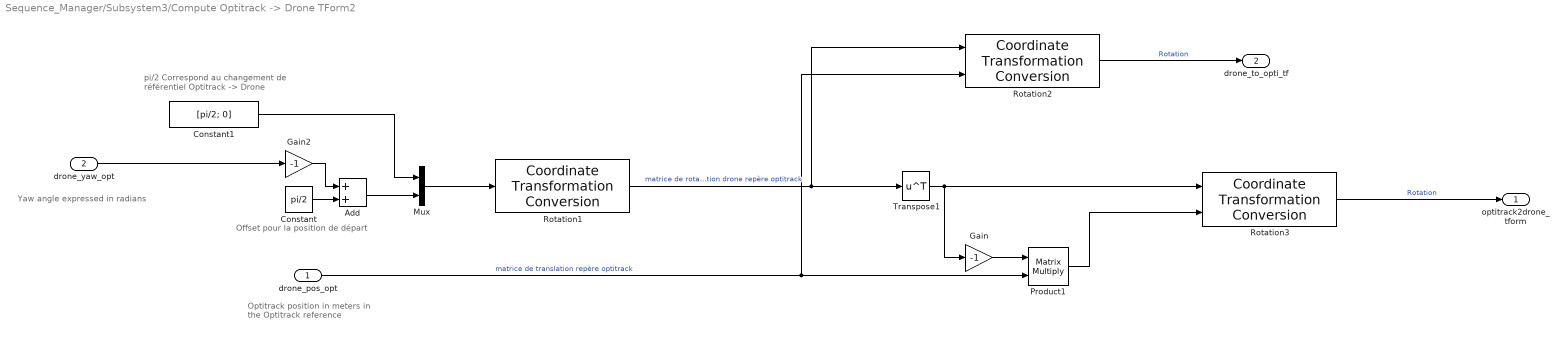
== system Sequence_Manager/Subsystem3/Compute Optitrack -> Drone TForm2 ==
  note: Yaw angle expressed in radians
  note: Offset pour la position de départ
  note: pi/2 Correspond au changement de référentiel Optitrack -> Drone
  note: Optitrack position in meters
      | in the Optitrack reference
  drone_pos_opt : Inport
  drone_yaw_opt : Inport  Port=2
  Add : Sum
  Constant : Constant  Value=pi/2
  Constant1 : Constant  Value=[pi/2; 0]
  Gain : Gain  Gain=-1
  Gain2 : Gain  Gain=-1
  Mux : Mux  Inputs=2
  Product1 : Product  Multiplication=Matrix(*)
  Rotation1 : robotcorelib/Coordinate Transformation Conversion  InputRepresentation=Euler Angles  InputEulerSequence=XYZ  ShowTrVecInputPort=off  OutputRepresentation=Rotation Matrix  OutputEulerSequence=ZYX  ShowTrVecOutputPort=off  SimulateUsing=Code generation
      settings: LibrarySourceBlock=uavutilslib/Coordinate Transformation Conversion
  Rotation2 : robotcorelib/Coordinate Transformation Conversion  InputRepresentation=Rotation Matrix  InputEulerSequence=XYZ  ShowTrVecInputPort=on  OutputRepresentation=Homogeneous Transformation  OutputEulerSequence=ZYX  ShowTrVecOutputPort=off  SimulateUsing=Code generation
      settings: LibrarySourceBlock=uavutilslib/Coordinate Transformation Conversion
  Rotation3 : robotcorelib/Coordinate Transformation Conversion  InputRepresentation=Rotation Matrix  InputEulerSequence=XYZ  ShowTrVecInputPort=on  OutputRepresentation=Homogeneous Transformation  OutputEulerSequence=ZYX  ShowTrVecOutputPort=off  SimulateUsing=Code generation
      settings: LibrarySourceBlock=uavutilslib/Coordinate Transformation Conversion
  Transpose1 : Math  Operator=transpose
  optitrack2drone_tform : Outport
  drone_to_opti_tf : Outport  Port=2
  wires:
  Add/1 -> Mux/2
  Transpose1/1 -> Rotation3/1, Gain/1
  Constant/1 -> Add/2
  Gain2/1 -> Add/1
  Product1/1 -> Rotation3/2
  Constant1/1 -> Mux/1
  Rotation1/1 -> Rotation2/1, Transpose1/1  "matrice de rotation drone repère optitrack"
  Gain/1 -> Product1/1
  Mux/1 -> Rotation1/1
  drone_pos_opt/1 -> Product1/2, Rotation2/2  "matrice de translation repère optitrack"
  drone_yaw_opt/1 -> Gain2/1
  Rotation3/1 -> optitrack2drone_tform/1  "Rotation"
  Rotation2/1 -> drone_to_opti_tf/1  "Rotation"

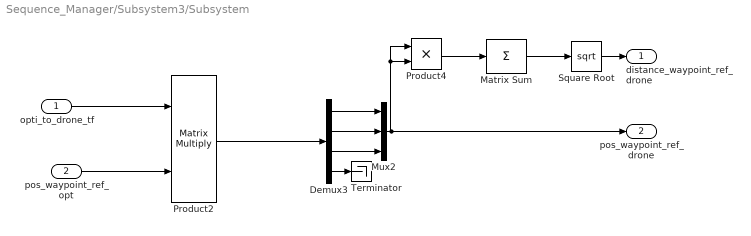
== system Sequence_Manager/Subsystem3/Subsystem ==
  opti_to_drone_tf : Inport
  pos_waypoint_ref_opt : Inport  Port=2
  Demux3 : Demux
  Matrix Sum : Sum  Inputs=+
  Mux2 : Mux  Inputs=3
  Product2 : Product  Multiplication=Matrix(*)
  Product4 : Product
  Square Root : Sqrt
  Terminator : Terminator
  distance_waypoint_ref_drone : Outport
  pos_waypoint_ref_drone : Outport  Port=2
  wires:
  Product2/1 -> Demux3/1
  opti_to_drone_tf/1 -> Product2/1
  Product4/1 -> Matrix Sum/1
  Demux3/2 -> Mux2/2
  Square Root/1 -> distance_waypoint_ref_drone/1
  Demux3/1 -> Mux2/1
  Mux2/1 -> pos_waypoint_ref_drone/1, Product4/1, Product4/2
  Matrix Sum/1 -> Square Root/1
  Demux3/3 -> Mux2/3
  Demux3/4 -> Terminator/1
  pos_waypoint_ref_opt/1 -> Product2/2
